simulink model "b"  (R2020a)
settings: Solver=VariableStepAuto  StartTime=0.0  StopTime=50  RelTol=1e-3
settings Model: Creator=hp  LastModifiedBy=hp

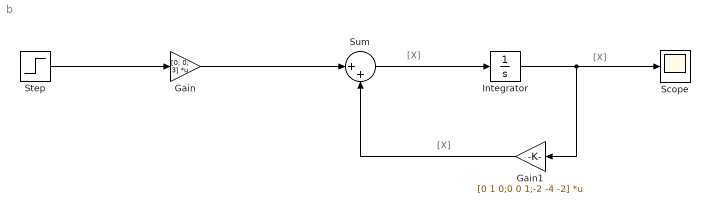
== system b ==
  note: [X]
  note: [X]
  note: [X]
  Gain : Gain  Gain=[0; 0; 3]  Multiplication=Matrix(K*u)
  Gain1 : Gain  Gain=[0 1 0;0 0 1;-2 -4 -2]  Multiplication=Matrix(K*u)
  Integrator : Integrator
  Scope : Scope
  Step : Step  SampleTime=0
  Sum : Sum  Inputs=|++
  wires:
  Sum/1 -> Integrator/1
  Gain/1 -> Sum/1
  Step/1 -> Gain/1
  Gain1/1 -> Sum/2
  Integrator/1 -> Gain1/1, Scope/1
